simulink model "CA1_model_change"  (R2023b)
settings: Solver=VariableStepAuto  StartTime=0.0  StopTime=200  RelTol=1e-3
values from neighbouring files (symbols this model uses):
  a1 = 0.22    [CA1_param.m]    (also in CA1_param_change.m)
  a11 = 20.4    [CA1_param_change.m]
  a2 = 6.1    [CA1_param.m]    (also in CA1_param_change.m)
  a22 = 6.4    [CA1_param_change.m]
  b0 = -0.5    [CA1_param.m]    (also in CA1_param_change.m)
  b00 = -2    [CA1_param_change.m]
  b1 = -1    [CA1_param.m]    (also in CA1_param_change.m)
  b11 = -5    [CA1_param_change.m]
  Gamma = diag([10000*g,10000*g,1000*g,1000*g,1000*g])    [CA1_param.m]    (also in CA1_param_change.m)
  t1 = T(2)    [CA1_param.m]    (also in CA1_param_change.m)
  t2 = T(3)    [CA1_param.m]    (also in CA1_param_change.m)
  tau = 1/10    (= 0.1)    [CA1_param.m]    (also in CA1_param_change.m)
settings Model: Creator=99551  LastModifiedBy=99551
settings DebuggingCC: UnconnectedInputMsg=warning  UnconnectedOutputMsg=warning  UnconnectedLineMsg=warning
settings ModelReferenceCC: EnableRefExpFcnMdlSchedulingChecks=on
settings RTWCC: DLArmComputeVersion=19.05

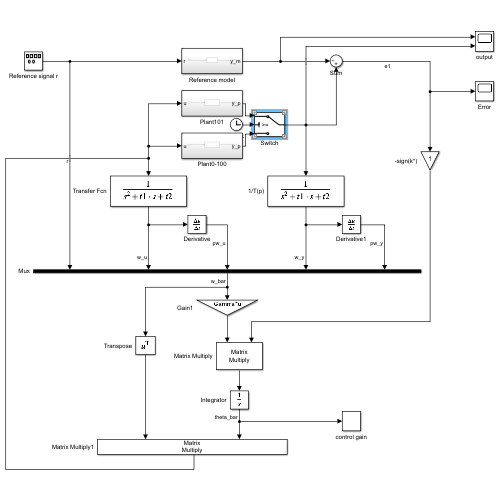
[thumbnail: Simulink's stored preview of the top-level diagram]
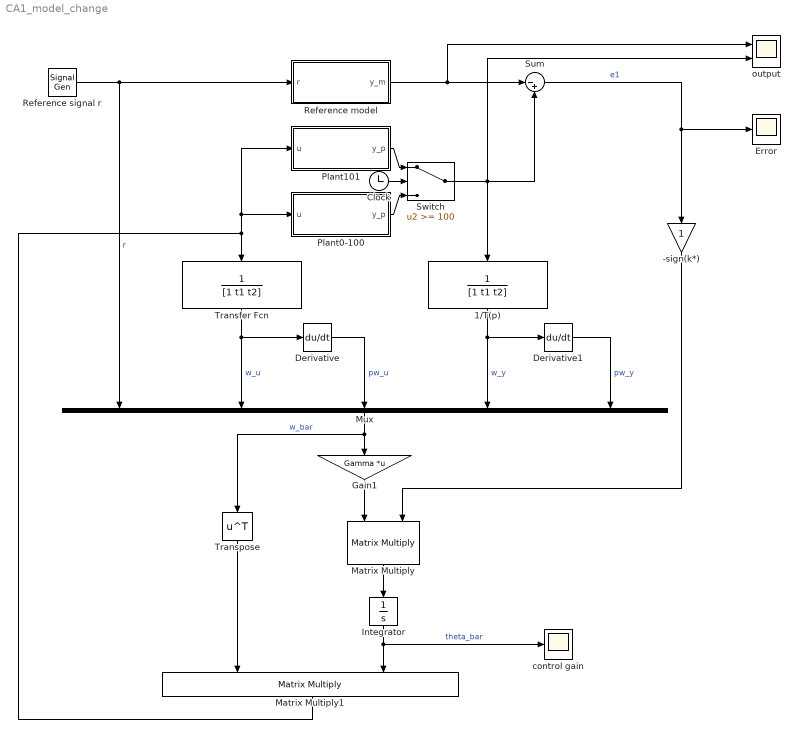
== system CA1_model_change ==
  -sign(k*) : Gain
  1/T(p) : TransferFcn  Denominator=[1 t1 t2]
  Clock : Clock
  Derivative : Derivative
  Derivative1 : Derivative
  Error : Scope
  Gain1 : Gain  Gain=Gamma  Multiplication=Matrix(K*u)
  Integrator : Integrator
  Matrix Multiply : Product  Multiplication=Matrix(*)
  Matrix Multiply1 : Product  Multiplication=Matrix(*)
  Mux : Mux  Inputs=5
  Plant0-100 : Subsystem
  Plant101 : Subsystem
  Reference model : Subsystem
  Reference signal r : SignalGenerator  WaveForm=square  Amplitude=10  Frequency=0.2
  Sum : Sum  Inputs=|-+
  Switch : Switch  Threshold=100  SaturateOnIntegerOverflow=off  InputSameDT=off
  Transfer Fcn : TransferFcn  Denominator=[1 t1 t2]
  Transpose : Math  Operator=transpose
  control gain : Scope
  output : Scope  NumInputPorts=2
  wires:
  Reference signal r/1 -> Mux/1, Reference model/1(r)  "r"
  Reference model/1(y_m) -> Sum/1, output/1
  Switch/1 -> output/2, 1/T(p)/1, Sum/2
  Sum/1 -> Error/1, -sign(k*)/1  "e1"
  Transfer Fcn/1 -> Mux/2, Derivative/1  "w_u"
  1/T(p)/1 -> Mux/4, Derivative1/1  "w_y"
  Derivative1/1 -> Mux/5  "pw_y"
  Derivative/1 -> Mux/3  "pw_u"
  Mux/1 -> Transpose/1, Gain1/1  "w_bar"
  Gain1/1 -> Matrix Multiply/1
  -sign(k*)/1 -> Matrix Multiply/2
  Matrix Multiply/1 -> Integrator/1
  Transpose/1 -> Matrix Multiply1/1
  Integrator/1 -> Matrix Multiply1/2, control gain/1  "theta_bar"
  Matrix Multiply1/1 -> Plant0-100/1(u), Plant101/1(u), Transfer Fcn/1
  Clock/1 -> Switch/2
  Plant101/1(y_p) -> Switch/1
  Plant0-100/1(y_p) -> Switch/3

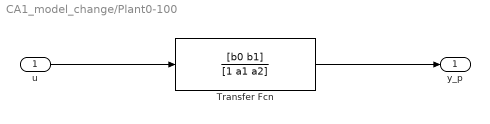
== system CA1_model_change/Plant0-100 ==
  u : Inport
  Transfer Fcn : TransferFcn  Numerator=[b0 b1]  Denominator=[1 a1 a2]
  y_p : Outport
  wires:
  u/1 -> Transfer Fcn/1
  Transfer Fcn/1 -> y_p/1

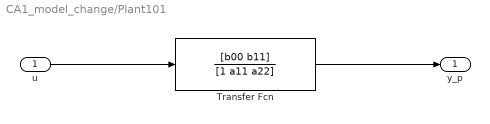
== system CA1_model_change/Plant101 ==
  u : Inport
  Transfer Fcn : TransferFcn  Numerator=[b00 b11]  Denominator=[1 a11 a22]
  y_p : Outport
  wires:
  u/1 -> Transfer Fcn/1
  Transfer Fcn/1 -> y_p/1

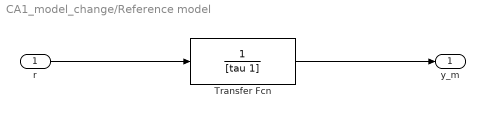
== system CA1_model_change/Reference model ==
  r : Inport
  Transfer Fcn : TransferFcn  Denominator=[tau 1]
  y_m : Outport
  wires:
  Transfer Fcn/1 -> y_m/1
  r/1 -> Transfer Fcn/1
